simulink model "spacecraft3"  (R2019b)
settings: Solver=VariableStepAuto  StartTime=0.0  StopTime=50  RelTol=1e-3
undefined symbols (not defined in the file or in its folder): DiscIntNeverNeededParam
libraries: simulink x5, vrlib x4, robotcorelib x2
settings Model: Creator=Tesla  LastModifiedBy=Tesla

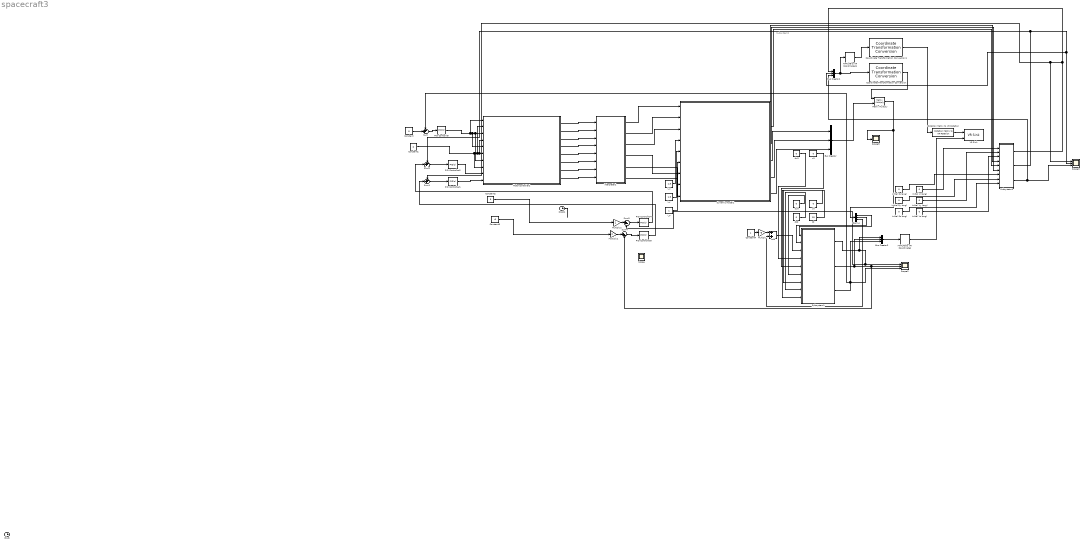
== system spacecraft3 ==
  note: Subsystem2
  Add : Sum
  Bus Creator : BusCreator  Inputs=3
  Bus Creator1 : BusCreator  Inputs=3
  Bus Creator2 : BusCreator  Inputs=3
  Clock : Clock
  Clock1 : Clock
  Constant : Constant  Value=5
  Constant1 : Constant  Value=0
  Constant2 : Constant  Value=5
  Constant3 : Constant  Value=-6
  Constant4 : Constant
  Coordinate Transformation Conversion : robotcorelib/Coordinate Transformation Conversion  InputRepresentation=Euler Angles  InputEulerSequence=XYZ  ShowTrVecInputPort=on  OutputRepresentation=Rotation Matrix  OutputEulerSequence=ZYX  ShowTrVecOutputPort=on  SimulateUsing=Interpreted execution
      settings: SourceProductBaseCode=RO
  Coordinate Transformation Conversion1 : robotcorelib/Coordinate Transformation Conversion  InputRepresentation=Euler Angles  InputEulerSequence=XYZ  ShowTrVecInputPort=on  OutputRepresentation=Rotation Matrix  OutputEulerSequence=ZYX  ShowTrVecOutputPort=on  SimulateUsing=Interpreted execution
      settings: SourceProductBaseCode=RO
  Demux : Demux  Outputs=3
  I_x : Constant  Value=1.5
  I_y : Constant  Value=1.5
  I_z : Constant
  Initial Rx(ang) : Constant  Value=0
  Initial Ry (ang) : Constant  Value=0
  Initial Rz (ang) : Constant  Value=0
  Initial Vx(ang) : Constant  Value=0
  Initial Vy (ang) : Constant  Value=0
  Initial Vz (ang) : Constant  Value=0
  MATLAB to VR Coordinates : vrlib/Utilities/MATLAB to VR Coordinates
      settings: SourceProductName=Simulink  SourceProductBaseCode=SL
  MATLAB to VR Coordinates1 : vrlib/Utilities/MATLAB to VR Coordinates
      settings: SourceProductName=Simulink  SourceProductBaseCode=SL
  Matrix Multiply : Product  Multiplication=Matrix(*)
  Motor controller1 : Subsystem
  Multiply : Gain  Gain=-5
  Multiply1 : Gain
  Multiply2 : Gain
  PID Controller : simulink/Continuous/PID Controller  Controller=PID  Form=Parallel  TimeDomain=Continuous-time  SampleTime=-1  IntegratorMethod=Forward Euler  FilterMethod=Forward Euler  ControllerParametersSource=internal  P=5  I=0  D=10  UseFilter=on  N=100  TunerSelectOption=Transfer Function Based (PID Tuner App)  InitialConditionSource=internal  InitialConditionForIntegrator=0  InitialConditionForFilter=0  DifferentiatorICPrevScaledInput=0  ExternalReset=none  TrackingMode=off  Kt=1  LimitOutput=on  UpperSaturationLimit=12  LowerSaturationLimit=0  LinearizeAsGain=on  AntiWindupMode=clamping  Kb=1  POutMin=[]  POutMax=[]  IOutMin=[]  IOutMax=[]  DOutMin=[]  DOutMax=[]  NOutMin=[]  NOutMax=[]  SumOutMin=[]  SumOutMax=[]  SaturationOutMin=[]  SaturationOutMax=[]  PParamMin=[]  PParamMax=[]  IParamMin=[]  IParamMax=[]  DParamMin=[]  DParamMax=[]  NParamMin=[]  NParamMax=[]  KbParamMin=[]  KbParamMax=[]  KtParamMin=[]  KtParamMax=[]  KbOutMin=[]  KbOutMax=[]  KtOutMin=[]  KtOutMax=[]  IntegratorOutMin=[]  IntegratorOutMax=[]  FilterOutMin=[]  FilterOutMax=[]  SumI1OutMin=[]  SumI1OutMax=[]  SumI2OutMin=[]  SumI2OutMax=[]  SumI3OutMin=[]  SumI3OutMax=[]  SumI4OutMin=[]  SumI4OutMax=[]  SumDOutMin=[]  SumDOutMax=[]  DifferentiatorOutMin=[]  DifferentiatorOutMax=[]  FilterDiffOutCoefMin=[]  FilterDiffOutCoefMax=[]  ReciprocalOutMin=[]  ReciprocalOutMax=[]  SumDenOutMin=[]  SumDenOutMax=[]  SumNumOutMin=[]  SumNumOutMax=[]  DivideOutMin=[]  DivideOutMax=[]  IntegratorContinuousStateAttributes=''  IntegratorStateMustResolveToSignalObject=off  IntegratorRTWStateStorageClass=Auto  FilterContinuousStateAttributes=''  FilterStateMustResolveToSignalObject=off  FilterRTWStateStorageClass=Auto  ParallelPVariant=InternalParameters  IdealPVariant=Disabled  IVariant=InternalParameters  DVariant=InternalParameters  IntegratorVariant=Continuous  SatVariant=Enabled  AWVariant=ContClampingParallel  PCopyVariant=Disabled  TRVariant=Disabled  FdbkBlocksVariant=Forward  IdealPFdbkVariant=Disabled  SatFdbkVariant=Disabled  DerivativeFilterVariant=ContFilter  NVariant=InternalParameters  NCopyVariant=Disabled  FilterICVariant=InternalICsFilter  IntegratorICVariant=InternalICs  ExternalResetVariant=Disabled  TRSumVariant=Passthrough  SumFdbkVariant=Disabled  SumVariant=Sum_PID
  PID Controller1 : simulink/Continuous/PID Controller  Controller=PID  Form=Parallel  TimeDomain=Continuous-time  SampleTime=-1  IntegratorMethod=Forward Euler  FilterMethod=Forward Euler  ControllerParametersSource=internal  P=-18  I=-3  D=-5  UseFilter=on  N=25  TunerSelectOption=Transfer Function Based (PID Tuner App)  InitialConditionSource=internal  InitialConditionForIntegrator=0  InitialConditionForFilter=0  DifferentiatorICPrevScaledInput=0  ExternalReset=none  TrackingMode=off  Kt=1  LimitOutput=on  UpperSaturationLimit=1.5  LowerSaturationLimit=-1.5  LinearizeAsGain=on  AntiWindupMode=clamping  Kb=1  POutMin=[]  POutMax=[]  IOutMin=[]  IOutMax=[]  DOutMin=[]  DOutMax=[]  NOutMin=[]  NOutMax=[]  SumOutMin=[]  SumOutMax=[]  SaturationOutMin=[]  SaturationOutMax=[]  PParamMin=[]  PParamMax=[]  IParamMin=[]  IParamMax=[]  DParamMin=[]  DParamMax=[]  NParamMin=[]  NParamMax=[]  KbParamMin=[]  KbParamMax=[]  KtParamMin=[]  KtParamMax=[]  KbOutMin=[]  KbOutMax=[]  KtOutMin=[]  KtOutMax=[]  IntegratorOutMin=[]  IntegratorOutMax=[]  FilterOutMin=[]  FilterOutMax=[]  SumI1OutMin=[]  SumI1OutMax=[]  SumI2OutMin=[]  SumI2OutMax=[]  SumI3OutMin=[]  SumI3OutMax=[]  SumI4OutMin=[]  SumI4OutMax=[]  SumDOutMin=[]  SumDOutMax=[]  DifferentiatorOutMin=[]  DifferentiatorOutMax=[]  FilterDiffOutCoefMin=[]  FilterDiffOutCoefMax=[]  ReciprocalOutMin=[]  ReciprocalOutMax=[]  SumDenOutMin=[]  SumDenOutMax=[]  SumNumOutMin=[]  SumNumOutMax=[]  DivideOutMin=[]  DivideOutMax=[]  IntegratorContinuousStateAttributes=''  IntegratorStateMustResolveToSignalObject=off  IntegratorRTWStateStorageClass=Auto  FilterContinuousStateAttributes=''  FilterStateMustResolveToSignalObject=off  FilterRTWStateStorageClass=Auto  ParallelPVariant=InternalParameters  IdealPVariant=Disabled  IVariant=InternalParameters  DVariant=InternalParameters  IntegratorVariant=Continuous  SatVariant=Enabled  AWVariant=ContClampingParallel  PCopyVariant=Disabled  TRVariant=Disabled  FdbkBlocksVariant=Forward  IdealPFdbkVariant=Disabled  SatFdbkVariant=Disabled  DerivativeFilterVariant=ContFilter  NVariant=InternalParameters  NCopyVariant=Disabled  FilterICVariant=InternalICsFilter  IntegratorICVariant=InternalICs  ExternalResetVariant=Disabled  TRSumVariant=Passthrough  SumFdbkVariant=Disabled  SumVariant=Sum_PID
  PID Controller2 : simulink/Continuous/PID Controller  Controller=PID  Form=Parallel  TimeDomain=Continuous-time  SampleTime=-1  IntegratorMethod=Forward Euler  FilterMethod=Forward Euler  ControllerParametersSource=internal  P=18  I=3  D=5  UseFilter=on  N=25  TunerSelectOption=Transfer Function Based (PID Tuner App)  InitialConditionSource=internal  InitialConditionForIntegrator=0  InitialConditionForFilter=0  DifferentiatorICPrevScaledInput=0  ExternalReset=none  TrackingMode=off  Kt=1  LimitOutput=on  UpperSaturationLimit=1.5  LowerSaturationLimit=-1.5  LinearizeAsGain=on  AntiWindupMode=clamping  Kb=1  POutMin=[]  POutMax=[]  IOutMin=[]  IOutMax=[]  DOutMin=[]  DOutMax=[]  NOutMin=[]  NOutMax=[]  SumOutMin=[]  SumOutMax=[]  SaturationOutMin=[]  SaturationOutMax=[]  PParamMin=[]  PParamMax=[]  IParamMin=[]  IParamMax=[]  DParamMin=[]  DParamMax=[]  NParamMin=[]  NParamMax=[]  KbParamMin=[]  KbParamMax=[]  KtParamMin=[]  KtParamMax=[]  KbOutMin=[]  KbOutMax=[]  KtOutMin=[]  KtOutMax=[]  IntegratorOutMin=[]  IntegratorOutMax=[]  FilterOutMin=[]  FilterOutMax=[]  SumI1OutMin=[]  SumI1OutMax=[]  SumI2OutMin=[]  SumI2OutMax=[]  SumI3OutMin=[]  SumI3OutMax=[]  SumI4OutMin=[]  SumI4OutMax=[]  SumDOutMin=[]  SumDOutMax=[]  DifferentiatorOutMin=[]  DifferentiatorOutMax=[]  FilterDiffOutCoefMin=[]  FilterDiffOutCoefMax=[]  ReciprocalOutMin=[]  ReciprocalOutMax=[]  SumDenOutMin=[]  SumDenOutMax=[]  SumNumOutMin=[]  SumNumOutMax=[]  DivideOutMin=[]  DivideOutMax=[]  IntegratorContinuousStateAttributes=''  IntegratorStateMustResolveToSignalObject=off  IntegratorRTWStateStorageClass=Auto  FilterContinuousStateAttributes=''  FilterStateMustResolveToSignalObject=off  FilterRTWStateStorageClass=Auto  ParallelPVariant=InternalParameters  IdealPVariant=Disabled  IVariant=InternalParameters  DVariant=InternalParameters  IntegratorVariant=Continuous  SatVariant=Enabled  AWVariant=ContClampingParallel  PCopyVariant=Disabled  TRVariant=Disabled  FdbkBlocksVariant=Forward  IdealPFdbkVariant=Disabled  SatFdbkVariant=Disabled  DerivativeFilterVariant=ContFilter  NVariant=InternalParameters  NCopyVariant=Disabled  FilterICVariant=InternalICsFilter  IntegratorICVariant=InternalICs  ExternalResetVariant=Disabled  TRSumVariant=Passthrough  SumFdbkVariant=Disabled  SumVariant=Sum_PID
  PID Controller3 : simulink/Continuous/PID Controller  Controller=PID  Form=Parallel  TimeDomain=Continuous-time  SampleTime=-1  IntegratorMethod=Forward Euler  FilterMethod=Forward Euler  ControllerParametersSource=internal  P=-0.11  I=-0.001  D=-0.09  UseFilter=on  N=25  TunerSelectOption=Transfer Function Based (PID Tuner App)  InitialConditionSource=internal  InitialConditionForIntegrator=0  InitialConditionForFilter=0  DifferentiatorICPrevScaledInput=0  ExternalReset=none  TrackingMode=off  Kt=1  LimitOutput=on  UpperSaturationLimit=1  LowerSaturationLimit=-1  LinearizeAsGain=off  AntiWindupMode=clamping  Kb=1  POutMin=[]  POutMax=[]  IOutMin=[]  IOutMax=[]  DOutMin=[]  DOutMax=[]  NOutMin=[]  NOutMax=[]  SumOutMin=[]  SumOutMax=[]  SaturationOutMin=[]  SaturationOutMax=[]  PParamMin=[]  PParamMax=[]  IParamMin=[]  IParamMax=[]  DParamMin=[]  DParamMax=[]  NParamMin=[]  NParamMax=[]  KbParamMin=[]  KbParamMax=[]  KtParamMin=[]  KtParamMax=[]  KbOutMin=[]  KbOutMax=[]  KtOutMin=[]  KtOutMax=[]  IntegratorOutMin=[]  IntegratorOutMax=[]  FilterOutMin=[]  FilterOutMax=[]  SumI1OutMin=[]  SumI1OutMax=[]  SumI2OutMin=[]  SumI2OutMax=[]  SumI3OutMin=[]  SumI3OutMax=[]  SumI4OutMin=[]  SumI4OutMax=[]  SumDOutMin=[]  SumDOutMax=[]  DifferentiatorOutMin=[]  DifferentiatorOutMax=[]  FilterDiffOutCoefMin=[]  FilterDiffOutCoefMax=[]  ReciprocalOutMin=[]  ReciprocalOutMax=[]  SumDenOutMin=[]  SumDenOutMax=[]  SumNumOutMin=[]  SumNumOutMax=[]  DivideOutMin=[]  DivideOutMax=[]  IntegratorContinuousStateAttributes=''  IntegratorStateMustResolveToSignalObject=off  IntegratorRTWStateStorageClass=Auto  FilterContinuousStateAttributes=''  FilterStateMustResolveToSignalObject=off  FilterRTWStateStorageClass=Auto  ParallelPVariant=InternalParameters  IdealPVariant=Disabled  IVariant=InternalParameters  DVariant=InternalParameters  IntegratorVariant=Continuous  SatVariant=Enabled  AWVariant=ContClampingParallel  PCopyVariant=Disabled  TRVariant=Disabled  FdbkBlocksVariant=Forward  IdealPFdbkVariant=Disabled  SatFdbkVariant=Disabled  DerivativeFilterVariant=ContFilter  NVariant=InternalParameters  NCopyVariant=Disabled  FilterICVariant=InternalICsFilter  IntegratorICVariant=InternalICs  ExternalResetVariant=Disabled  TRSumVariant=Passthrough  SumFdbkVariant=Disabled  SumVariant=Sum_PID
  PID Controller4 : simulink/Continuous/PID Controller  Controller=PID  Form=Parallel  TimeDomain=Continuous-time  SampleTime=-1  IntegratorMethod=Forward Euler  FilterMethod=Forward Euler  ControllerParametersSource=internal  P=0.11  I=0.001  D=0.09  UseFilter=on  N=25  TunerSelectOption=Transfer Function Based (PID Tuner App)  InitialConditionSource=internal  InitialConditionForIntegrator=0  InitialConditionForFilter=0  DifferentiatorICPrevScaledInput=0  ExternalReset=none  TrackingMode=off  Kt=1  LimitOutput=on  UpperSaturationLimit=1  LowerSaturationLimit=-1  LinearizeAsGain=off  AntiWindupMode=clamping  Kb=1  POutMin=[]  POutMax=[]  IOutMin=[]  IOutMax=[]  DOutMin=[]  DOutMax=[]  NOutMin=[]  NOutMax=[]  SumOutMin=[]  SumOutMax=[]  SaturationOutMin=[]  SaturationOutMax=[]  PParamMin=[]  PParamMax=[]  IParamMin=[]  IParamMax=[]  DParamMin=[]  DParamMax=[]  NParamMin=[]  NParamMax=[]  KbParamMin=[]  KbParamMax=[]  KtParamMin=[]  KtParamMax=[]  KbOutMin=[]  KbOutMax=[]  KtOutMin=[]  KtOutMax=[]  IntegratorOutMin=[]  IntegratorOutMax=[]  FilterOutMin=[]  FilterOutMax=[]  SumI1OutMin=[]  SumI1OutMax=[]  SumI2OutMin=[]  SumI2OutMax=[]  SumI3OutMin=[]  SumI3OutMax=[]  SumI4OutMin=[]  SumI4OutMax=[]  SumDOutMin=[]  SumDOutMax=[]  DifferentiatorOutMin=[]  DifferentiatorOutMax=[]  FilterDiffOutCoefMin=[]  FilterDiffOutCoefMax=[]  ReciprocalOutMin=[]  ReciprocalOutMax=[]  SumDenOutMin=[]  SumDenOutMax=[]  SumNumOutMin=[]  SumNumOutMax=[]  DivideOutMin=[]  DivideOutMax=[]  IntegratorContinuousStateAttributes=''  IntegratorStateMustResolveToSignalObject=off  IntegratorRTWStateStorageClass=Auto  FilterContinuousStateAttributes=''  FilterStateMustResolveToSignalObject=off  FilterRTWStateStorageClass=Auto  ParallelPVariant=InternalParameters  IdealPVariant=Disabled  IVariant=InternalParameters  DVariant=InternalParameters  IntegratorVariant=Continuous  SatVariant=Enabled  AWVariant=ContClampingParallel  PCopyVariant=Disabled  TRVariant=Disabled  FdbkBlocksVariant=Forward  IdealPFdbkVariant=Disabled  SatFdbkVariant=Disabled  DerivativeFilterVariant=ContFilter  NVariant=InternalParameters  NCopyVariant=Disabled  FilterICVariant=InternalICsFilter  IntegratorICVariant=InternalICs  ExternalResetVariant=Disabled  TRSumVariant=Passthrough  SumFdbkVariant=Disabled  SumVariant=Sum_PID
  Rotation Matrix to VR Rotation : vrlib/Utilities/Rotation Matrix to VR Rotation  maxzero=1e-12
      settings: SourceProductName=Simulink  SourceProductBaseCode=SL
  Scope : Scope  NumInputPorts=2
  Scope2 : Scope  NumInputPorts=3
  Scope3 : Scope  NumInputPorts=3
  Scope5 : Scope
  Subsystem1 : Subsystem
  Subsystem3 : Subsystem
  Sum : Sum  Inputs=-+|
  Sum1 : Sum  Inputs=-+|
  Sum2 : Sum  Inputs=-+|
  Sum3 : Sum  Inputs=|+-
  Sum4 : Sum  Inputs=|+-
  VR Sink : vrlib/VR Sink  InstantiateOnLoad=on  SampleTime=0.02  ViewEnable=on  RemoteChange=off  RemoteView=off  FieldsWritten=vehicle.rotation.4.1.1.double#vehicle.translation.3.1.1.double  WorldFileName=advance.wrl  AutoView=off  VideoDimensions=[200 320]  AllowVariableSize=off  FigureProperties="{'Position', 'Name', 'Viewpoint', 'CameraBound', 'CameraDirection', 'CameraPosition', 'CameraUpVector', 'ZoomFactor', 'Antialiasing', 'Headlight', 'Lighting', 'NavPanel', 'Sound', 'StatusBar', 'Stereo3D', 'Stereo3DCameraOffset', 'Stereo3DHIT', 'ToolBar', 'Textures', 'Transparency', 'Triad', 'Wireframe', 'NavZones', 'NavMode', 'NavSpeed', 'CaptureFileFormat', 'CaptureFileName', 'Record2DCompressMethod', 'Record2DCompressQuality', 'Record2D', 'Record2DFileName', 'Record2DFPS'; [1.0000000000000000e+00   7.6000000000000000e+01   1.9200000000000000e+03   9.1300000000000000e+02], '', '_untitled_1', 'on', [5.7402643959969801e-02  -3.3701133849065446e-01  -9.3974905916161466e-01], [9.6333963950548984e-01  -1.9685989701925708e+00   3.7041274962465813e+00], [5.8037188612519774e-02   9.4083573683776467e-01  -3.3385595850140015e-01], [1.0000000000000000e+00], 'off', 'on', 'on', 'halfbar', 'on', 'on', 'off', [1.0000000149011612e-01], [0.0000000000000000e+00], 'on', 'on', 'on', 'none', 'off', 'off', 'examine', 'normal', 'tif', '%f_anim_%n.tif', 'auto', [7.5000000000000000e+01], 'off', '%f_anim_%n.avi', 'auto'}"
      settings: SourceProductName=Simulink
  dx0 : Constant  Value=0
  dy0 : Constant  Value=0
  dynamic model1 : MATLAB Function  TreatAsAtomicUnit=on
  dz0 : Constant  Value=0
  interpreter1 : MATLAB Function  TreatAsAtomicUnit=on
  x0 : Constant  Value=0
  y0 : Constant  Value=0
  z0 : Constant  Value=15
  wires:
  dynamic model1/1(ANGx) -> Subsystem3/4(In3)
  Initial Vy (ang)/1 -> Subsystem3/2(In2)
  interpreter1/6(Thrust_z) -> dynamic model1/9(Thrust_z)
  interpreter1/3(tau_z) -> dynamic model1/3(tau_z)
  Initial Rz (ang)/1 -> Subsystem3/9(In8)
  interpreter1/4(Thrust_x) -> dynamic model1/7(Thrust_x)
  interpreter1/2(tau_y) -> dynamic model1/2(tau_y)
  interpreter1/5(Thrust_y) -> dynamic model1/8(Thrust_y)
  I_x/1 -> dynamic model1/4(I_x)
  dynamic model1/3(ANGz) -> Subsystem3/6(In5)
  I_y/1 -> dynamic model1/5(I_y)
  Initial Ry (ang)/1 -> Subsystem3/8(In7)
  interpreter1/1(tau_x) -> dynamic model1/1(tau_x)
  Initial Vz (ang)/1 -> Subsystem3/3(Input)
  I_z/1 -> dynamic model1/6(I_z)
  dynamic model1/2(ANGy) -> Subsystem3/5(In4)
  Initial Vx(ang)/1 -> Subsystem3/1(In1)
  Initial Rx(ang)/1 -> Subsystem3/7(In6)
  dynamic model1/6(accz) -> Bus Creator/3
  Subsystem3/3(Out3) -> Bus Creator1/3, Scope3/3
  Demux/1 -> Subsystem1/1(In1)
  MATLAB to VR Coordinates/1 -> VR Sink/2
  Coordinate Transformation Conversion/1 -> Matrix Multiply/1
  z0/1 -> Subsystem1/9(In9)
  dz0/1 -> Subsystem1/8(In8)
  x0/1 -> Subsystem1/5(In5)
  dx0/1 -> Subsystem1/4(In4)
  dy0/1 -> Subsystem1/6(In6)
  dynamic model1/5(accy) -> Bus Creator/2
  Bus Creator2/1 -> MATLAB to VR Coordinates/1
  Subsystem3/1(Out1) -> Sum1/1, Scope3/1, Bus Creator1/1
  Subsystem3/2(Out2) -> Bus Creator1/2, Scope3/2, Sum2/1
  Rotation Matrix to VR Rotation/1 -> VR Sink/1
  dynamic model1/4(accx) -> Bus Creator/1
  y0/1 -> Subsystem1/7(In7)
  Subsystem1/3(Out3) -> Scope2/3, Sum/1, Bus Creator2/3
  Demux/2 -> Subsystem1/2(In2)
  Bus Creator/1 -> Matrix Multiply/2
  Matrix Multiply/1 -> Scope5/1, Demux/1
  Coordinate Transformation Conversion1/1 -> Rotation Matrix to VR Rotation/1
  Bus Creator1/1 -> Coordinate Transformation Conversion/1, MATLAB to VR Coordinates1/1
  Demux/3 -> Add/2
  Motor controller1/1("E8 ") -> interpreter1/1(E8)
  Motor controller1/2(E1) -> interpreter1/2(E1)
  Motor controller1/3(E2) -> interpreter1/3(E2)
  Motor controller1/4(E3) -> interpreter1/4(E3)
  Motor controller1/5(E4) -> interpreter1/5(E4)
  Motor controller1/6(E5) -> interpreter1/6(E5)
  Motor controller1/7(E6) -> interpreter1/7(E6)
  Motor controller1/8(E7) -> interpreter1/8(E7)
  Constant1/1 -> Motor controller1/8(alpha_4), Motor controller1/2(alpha_1), Motor controller1/4(alpha_2), Motor controller1/6(alpha_3)
  MATLAB to VR Coordinates1/1 -> Coordinate Transformation Conversion1/1
  PID Controller/1 -> Motor controller1/7(Tau_4), Motor controller1/3(Tau_2), Motor controller1/5(Tau_3), Motor controller1/1("Tau_1 ")
  Constant/1 -> Sum/2
  Sum/1 -> PID Controller/1
  Sum1/1 -> PID Controller1/1
  PID Controller1/1 -> Motor controller1/10(Rot_X)
  Sum2/1 -> PID Controller2/1
  PID Controller2/1 -> Motor controller1/9(Rot_Y)
  PID Controller3/1 -> Sum1/2
  Multiply2/1 -> Sum3/1
  Multiply1/1 -> Sum4/1
  Sum3/1 -> PID Controller4/1
  PID Controller4/1 -> Sum2/2
  Subsystem1/1(Out1) -> Bus Creator2/1, Scope2/1, Sum3/2
  Sum4/1 -> PID Controller3/1
  Subsystem1/2(Out2) -> Bus Creator2/2, Scope2/2, Sum4/2
  Clock1/1 -> ?
  Constant2/1 -> Multiply2/1
  Constant3/1 -> Multiply1/1
  Constant4/1 -> Multiply/1
  Multiply/1 -> Add/1
  Add/1 -> Subsystem1/3(In3)

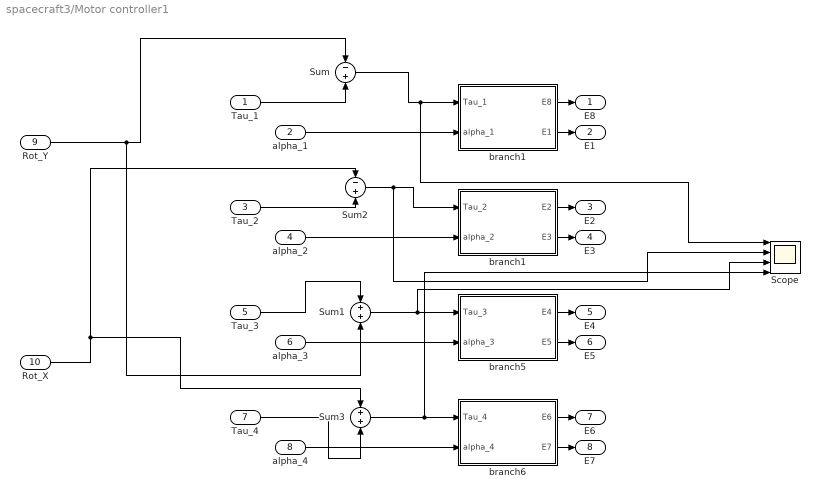
== system spacecraft3/Motor controller1 ==
  "Tau_1 " : Inport
  alpha_1 : Inport  Port=2
  Tau_2 : Inport  Port=3
  alpha_2 : Inport  Port=4
  Tau_3 : Inport  Port=5
  alpha_3 : Inport  Port=6
  Tau_4 : Inport  Port=7
  alpha_4 : Inport  Port=8
  Rot_Y : Inport  Port=9
  Rot_X : Inport  Port=10
  Scope : Scope  NumInputPorts=4
  Sum : Sum  Inputs=-|+
  Sum1 : Sum  Inputs=+|+
  Sum2 : Sum  Inputs=-|+
  Sum3 : Sum  Inputs=+|+
  branch1 : MATLAB Function  TreatAsAtomicUnit=on
  "branch1 " : MATLAB Function  TreatAsAtomicUnit=on
  branch5 : MATLAB Function  TreatAsAtomicUnit=on
  branch6 : MATLAB Function  TreatAsAtomicUnit=on
  "E8 " : Outport
  E1 : Outport  Port=2
  E2 : Outport  Port=3
  E3 : Outport  Port=4
  E4 : Outport  Port=5
  E5 : Outport  Port=6
  E6 : Outport  Port=7
  E7 : Outport  Port=8
  wires:
  Sum/1 -> Scope/1, "branch1 "/1(Tau_1)
  Sum3/1 -> Scope/4, branch6/1(Tau_4)
  Rot_X/1 -> Sum2/1, Sum3/1
  Tau_4/1 -> Sum3/2
  Tau_2/1 -> Sum2/2
  Tau_3/1 -> Sum1/1
  Sum2/1 -> Scope/2, branch1/1(Tau_2)
  alpha_2/1 -> branch1/2(alpha_2)
  branch6/1(E6) -> E6/1
  Rot_Y/1 -> Sum1/2, Sum/1
  Sum1/1 -> Scope/3, branch5/1(Tau_3)
  "Tau_1 "/1 -> Sum/2
  alpha_4/1 -> branch6/2(alpha_4)
  alpha_1/1 -> "branch1 "/2(alpha_1)
  alpha_3/1 -> branch5/2(alpha_3)
  branch1/2(E3) -> E3/1
  branch1/1(E2) -> E2/1
  "branch1 "/1(E8) -> "E8 "/1
  "branch1 "/2(E1) -> E1/1
  branch5/2(E5) -> E5/1
  branch6/2(E7) -> E7/1
  branch5/1(E4) -> E4/1

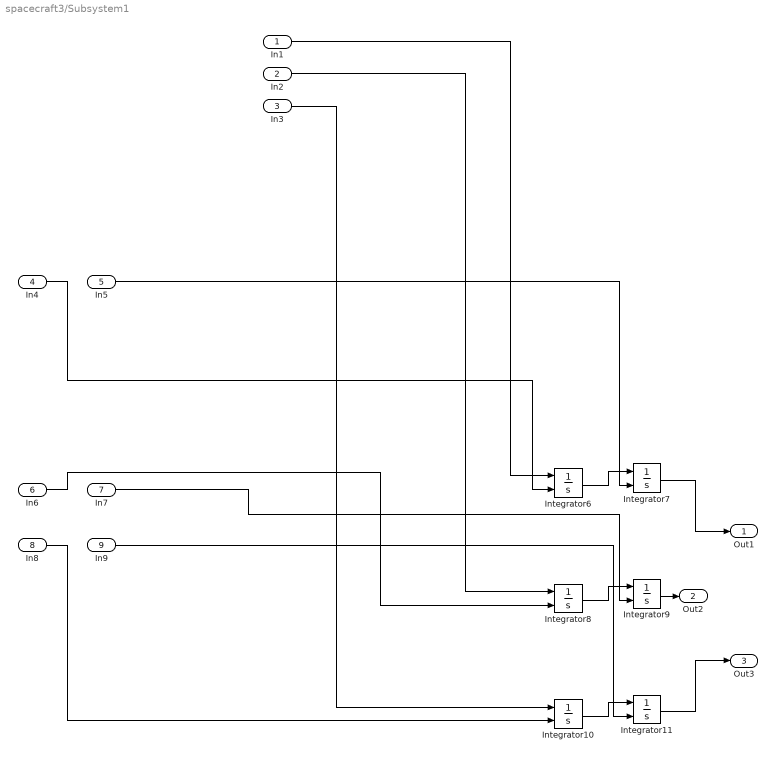
== system spacecraft3/Subsystem1 ==
  In1 : Inport
  In2 : Inport  Port=2
  In3 : Inport  Port=3
  In4 : Inport  Port=4
  In5 : Inport  Port=5
  In6 : Inport  Port=6
  In7 : Inport  Port=7
  In8 : Inport  Port=8
  In9 : Inport  Port=9
  Integrator{6..11} (6 alike) : Integrator  InitialConditionSource=external
  Out1 : Outport
  Out2 : Outport  Port=2
  Out3 : Outport  Port=3
  wires:
  In7/1 -> Integrator9/2
  Integrator10/1 -> Integrator11/1
  In6/1 -> Integrator8/2
  In4/1 -> Integrator6/2
  In9/1 -> Integrator11/2
  Integrator6/1 -> Integrator7/1
  In3/1 -> Integrator10/1
  Integrator9/1 -> Out2/1
  In8/1 -> Integrator10/2
  Integrator8/1 -> Integrator9/1
  In1/1 -> Integrator6/1
  In2/1 -> Integrator8/1
  Integrator7/1 -> Out1/1
  In5/1 -> Integrator7/2
  Integrator11/1 -> Out3/1

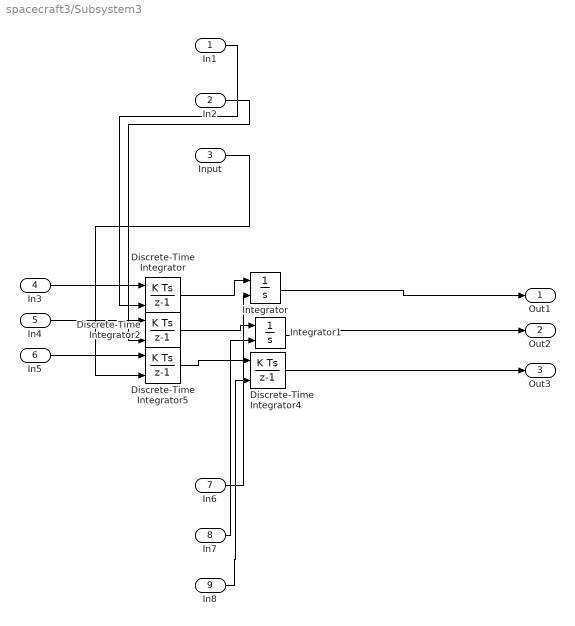
== system spacecraft3/Subsystem3 ==
  In1 : Inport
  In2 : Inport  Port=2
  Input : Inport  Port=3
  In3 : Inport  Port=4
  In4 : Inport  Port=5
  In5 : Inport  Port=6
  In6 : Inport  Port=7
  In7 : Inport  Port=8
  In8 : Inport  Port=9
  Discrete-Time Integrator : DiscreteIntegrator  InitialConditionSource=external  SampleTime=0.01  ICPrevOutput=DiscIntNeverNeededParam  ICPrevScaledInput=DiscIntNeverNeededParam
  Discrete-Time Integrator2 : DiscreteIntegrator  InitialConditionSource=external  SampleTime=-1  ICPrevOutput=DiscIntNeverNeededParam  ICPrevScaledInput=DiscIntNeverNeededParam
  Discrete-Time Integrator4 : DiscreteIntegrator  InitialConditionSource=external  SampleTime=-1  ICPrevOutput=DiscIntNeverNeededParam  ICPrevScaledInput=DiscIntNeverNeededParam
  Discrete-Time Integrator5 : DiscreteIntegrator  InitialConditionSource=external  SampleTime=-1  ICPrevOutput=DiscIntNeverNeededParam  ICPrevScaledInput=DiscIntNeverNeededParam
  Integrator : Integrator  InitialConditionSource=external
  Integrator1 : Integrator  InitialConditionSource=external
  Out1 : Outport
  Out2 : Outport  Port=2
  Out3 : Outport  Port=3
  wires:
  In5/1 -> Discrete-Time Integrator5/1
  Discrete-Time Integrator4/1 -> Out3/1
  Discrete-Time Integrator2/1 -> Integrator1/1
  In6/1 -> Integrator/2
  Input/1 -> Discrete-Time Integrator5/2
  Discrete-Time Integrator5/1 -> Discrete-Time Integrator4/1
  In8/1 -> Discrete-Time Integrator4/2
  Discrete-Time Integrator/1 -> Integrator/1
  Integrator/1 -> Out1/1
  Integrator1/1 -> Out2/1
  In4/1 -> Discrete-Time Integrator2/1
  In7/1 -> Integrator1/2
  In2/1 -> Discrete-Time Integrator2/2
  In3/1 -> Discrete-Time Integrator/1
  In1/1 -> Discrete-Time Integrator/2

== matlab function spacecraft3/Motor controller1/branch1 ==
  data: Tau_2 input; E2 output; alpha_2 input; E3 output
function[E2, E3] = fcn(Tau_2, alpha_2)
    E2 = (Tau_2 - (alpha_2*Tau_2))*0.5;
    E3 = (Tau_2 + (alpha_2*Tau_2))*0.5;
end

== matlab function spacecraft3/Motor controller1/branch1  ==
  data: Tau_1 input; E8 output; alpha_1 input; E1 output
function[E8, E1] = fcn(Tau_1, alpha_1)
    E8 = (Tau_1 - (alpha_1*Tau_1))*0.5;
    E1 = (Tau_1 + (alpha_1*Tau_1))*0.5;
end

== matlab function spacecraft3/Motor controller1/branch5 ==
  data: Tau_3 input; E4 output; alpha_3 input; E5 output
function[E4, E5] = fcn(Tau_3, alpha_3)
    E4 = (Tau_3 - (alpha_3*Tau_3))*0.5;
    E5 = (Tau_3 + (alpha_3*Tau_3))*0.5;
end

== matlab function spacecraft3/Motor controller1/branch6 ==
  data: Tau_4 input; E6 output; alpha_4 input; E7 output
function[E6, E7] = fcn(Tau_4, alpha_4)
    E6 = (Tau_4 - (alpha_4*Tau_4))*0.5;
    E7 = (Tau_4 + (alpha_4*Tau_4))*0.5;
end

== matlab function spacecraft3/dynamic model1 ==
  data: tau_x input; ANGx output; tau_y input; tau_z input; I_x input; I_y input; I_z input; Thrust_x input; Thrust_y input; Thrust_z input; ANGy output; ANGz output; accx output; accy output; accz output
function [ANGx, ANGy, ANGz, accx ,accy, accz] = fcn(tau_x, tau_y, tau_z, I_x, I_y, I_z,Thrust_x,Thrust_y,Thrust_z)

mass = 1;
g = -5;
ANG = [tau_x/I_x;tau_y/I_y;tau_z/I_z];

ANGx = ANG(1);
ANGy = ANG(2);
ANGz = ANG(3);

acc = [(Thrust_x/mass);(Thrust_y/mass);(Thrust_z/mass)];
accx = acc(1);
accy = acc(2);
accz = acc(3);
end

== matlab function spacecraft3/interpreter1 ==
  data: E8 input; tau_x output; E1 input; E2 input; E3 input; E4 input; E5 input; E6 input; E7 input; tau_y output; tau_z output; Thrust_x output; Thrust_y output; Thrust_z output
function [tau_x, tau_y, tau_z, Thrust_x, Thrust_y, Thrust_z] = fcn(E8, E1, E2, E3, E4, E5, E6, E7)

tau_x = ((E2+E3)-(E6+E7)) + 0.1*((E1+E4)-(E5+E8));
tau_y = ((E4+E5)-(E1+E8)) + 0.1*((E3+E6)-(E2+E7));
tau_z = (0.1*(E2+E6+E8+E4) - 0.1*(E3+E7+E1+E5));

Thrust_z = E1+E2+E3+E4+E5+E6+E7+E8;
Thrust_y = (0.1*(E5+E8)) - (0.1*(E4+E1));
Thrust_x = (0.1*(E3+E6)) - (0.1*(E2+E7));

end
